simulink model "Test3"  (R2017b)
settings: Solver=ode23tb  StartTime=0.0  StopTime=6  MaxStep=1e-4  RelTol=1e-3
libraries: powerlib x4
settings Model: Creator=80573  LastModifiedBy=80573

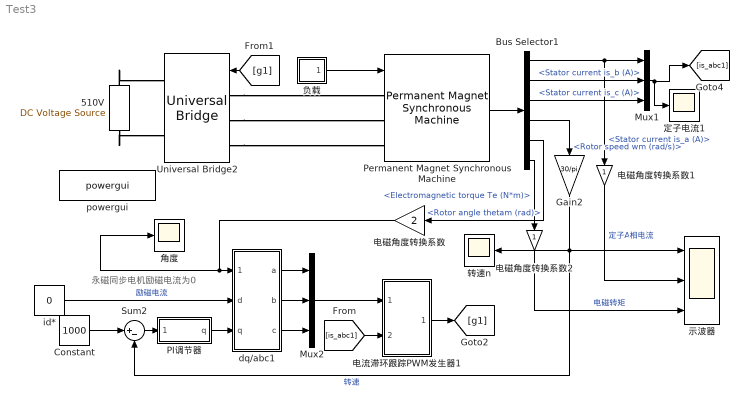
== system Test3 ==
  note: 永磁同步电机励磁电流为0
  510V : powerlib/Electrical Sources/DC Voltage Source  Amplitude=800  Measurements=None
  Bus Selector1 : BusSelector  OutputSignals=Stator current is_a (A),Stator current is_b (A),Stator current is_c (A),Rotor speed wm (rad/s),Rotor angle thetam (rad),Electromagnetic torque Te (N*m)
  Constant : Constant  Value=1000
  Gain2 : Gain  Gain=30/pi
  Mux1 : Mux  Inputs=3
  Mux2 : Mux  Inputs=3
  PI调节器 : Subsystem
  Permanent Magnet Synchronous Machine : powerlib/Machines/Permanent Magnet Synchronous Machine  NbPhases=3  FluxDistribution=Sinusoidal  RotorType=Salient-pole  MechanicalLoad=Torque Tm  PresetModel=No  ShowDetailedParameters=on  MeasurementBus=off  Resistance=0.00275  Inductance=8.5e-3  dqInductances=[0.000085 0.000085]  La=0.02682  MachineConstant=Flux linkage established by magnets (V.s)  Flux=1  VoltageCst=362.7599  TorqueCst=3  Flat=120  Mechanical=[1 0.008 2 0]  PolePairs=2  InitialConditions=[0,0, 0,0]  InitialConditions5ph=[0 0 0 0 0 0]  TsPowergui=0  TsBlock=-1  RefAngle=Aligned with phase A axis (original Park)
      settings: SourceProductName=Simscape Power Systems
  Sum2 : Sum  Inputs=|+-
  Universal Bridge2 : powerlib/Power Electronics/Universal Bridge  Arms=3  SnubberResistance=1e5  SnubberCapacitance=inf  Device=IGBT / Diodes  Ron=1e-3  Lon=0  ForwardVoltages="[  0  0  ]"  ForwardVoltage=0  GTOparameters=[ 10e-6 , 20e-6 ]  IGBTparameters=[ 1e-6 , 2e-6 ]  Measurements=None  Measurements_2=None  converterType=Rectifier
  dq/abc1 : Subsystem
  id* : Constant  Value=0
  powergui : powerlib/powergui  SimulationMode=Discrete  SampleTime=0.00001  frequency=50  Iterations=50  frequencyindice=0  Pbase=100e6  ErrMax=1e-4  UnitsV=kV  UnitsW=MW  buscounter=0  FunctionMessages=off  echomessages=off  EnableUseOfTLC=off  CurrentSourceSwitches=off  DisableSnubberDevices=off  DisableRonSwitches=off  DisableVfSwitches=off  DisplayEquations=off  SolverType=Tustin/Backward Euler (TBE)  Interpol=off  ExternalGateDelay=off  methode=off  Ts=100  x0status=zero  SPID=on  SwTol=0  HookPort=off  RestoreLinks=warning  ResistiveCurrentMeasurement=off  Frange=[0:2:500]  Ylog=off  Xlog=on  ShowGrid=off  save=off  variable=ZData  structure=0  ZoomFFT=on  StartTime=0.0  cycles=1  DisplayStyle=1  fundamental=60  FreqAxis=off  MaxFrequency=1000  frequencyindicesteady=1  RmsSteady=1  display=off
  定子电流1 : Scope
  电流滞环跟踪PWM发生器1 : Subsystem
  电磁角度转换系数 : Gain  Gain=2
  电磁角度转换系数1 : Gain
  电磁角度转换系数2 : Gain
  示波器 : Scope  NumInputPorts=3
  角度 : Scope
  负载 : Subsystem
  转速n : Scope
  wires:
  Bus Selector1/3 -> Mux1/3  "<Stator current is_c (A)>"
  Mux1/1 -> [is_abc1], 定子电流1/1
  Bus Selector1/5 -> 电磁角度转换系数/1  "<Rotor angle thetam (rad)>"
  dq/abc1/3(c) -> Mux2/3
  [is_abc1] -> 电流滞环跟踪PWM发生器1/2(Iabc)
  电流滞环跟踪PWM发生器1/1(pulse) -> [g1]
  PI调节器/1(q) -> dq/abc1/3(q)
  Gain2/1 -> 示波器/1, Sum2/2, 转速n/1  "转速"
  [g1] -> Universal Bridge2/1
  Bus Selector1/6 -> 电磁角度转换系数2/1  "<Electromagnetic torque Te (N*m)>"
  dq/abc1/2(b) -> Mux2/2
  电磁角度转换系数2/1 -> 示波器/3  "电磁转矩"
  电磁角度转换系数1/1 -> 示波器/2  "定子A相电流"
  Mux2/1 -> 电流滞环跟踪PWM发生器1/1(Iabc*)
  Bus Selector1/1 -> Mux1/1, 电磁角度转换系数1/1  "<Stator current is_a (A)>"
  Permanent Magnet Synchronous Machine/1 -> Bus Selector1/1
  id*/1 -> dq/abc1/2(d)  "励磁电流"
  电磁角度转换系数/1 -> 角度/1, dq/abc1/1(theta)
  Bus Selector1/4 -> Gain2/1  "<Rotor speed wm (rad/s)>"
  Sum2/1 -> PI调节器/1("  ")
  负载/1(TL) -> Permanent Magnet Synchronous Machine/1
  Constant/1 -> Sum2/1
  dq/abc1/1(a) -> Mux2/1
  Bus Selector1/2 -> Mux1/2  "<Stator current is_b (A)>"
  connections:
  510V/RConn1 -- Universal Bridge2/RConn1
  Universal Bridge2/LConn1 -- Permanent Magnet Synchronous Machine/LConn1
  Universal Bridge2/LConn3 -- Permanent Magnet Synchronous Machine/LConn3
  510V/LConn1 -- Universal Bridge2/RConn2
  Universal Bridge2/LConn2 -- Permanent Magnet Synchronous Machine/LConn2

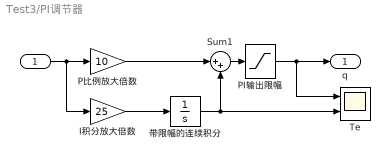
== system Test3/PI调节器 ==
  "  " : Inport
  I积分放大倍数 : Gain  Gain=25
  PI输出限幅 : Saturate  UpperLimit=500  LowerLimit=-500
  P比例放大倍数 : Gain  Gain=10
  Sum1 : Sum  Inputs=|++
  Te : Scope  NumInputPorts=2
  带限幅的连续积分 : Integrator  LimitOutput=on  UpperSaturationLimit=510  LowerSaturationLimit=-510
  q : Outport
  wires:
  Sum1/1 -> PI输出限幅/1
  PI输出限幅/1 -> q/1, Te/1
  P比例放大倍数/1 -> Sum1/1
  I积分放大倍数/1 -> 带限幅的连续积分/1
  带限幅的连续积分/1 -> Te/2, Sum1/2
  "  "/1 -> I积分放大倍数/1, P比例放大倍数/1

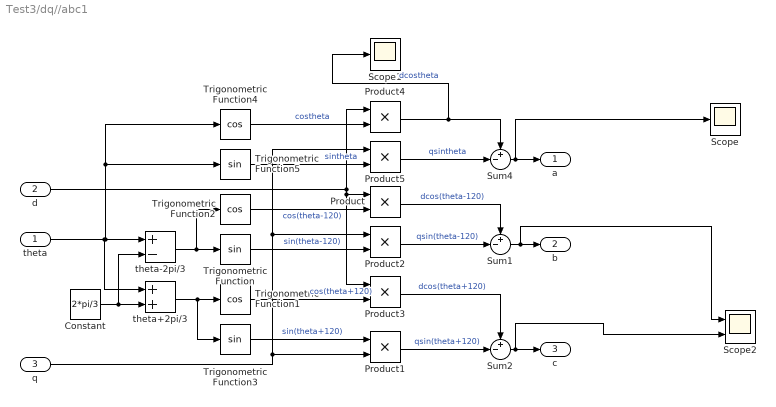
== system Test3/dq//abc1 ==
  theta : Inport
  d : Inport  Port=2
  q : Inport  Port=3
  Constant : Constant  Value=2*pi/3
  Product{,1..5} (6 alike) : Product
  Scope : Scope
  Scope1 : Scope
  Scope2 : Scope  NumInputPorts=2
  Sum1 : Sum  Inputs=+-|
  Sum2 : Sum  Inputs=+-|
  Sum4 : Sum  Inputs=+-|
  Trigonometric Function : Trigonometry
  Trigonometric Function1 : Trigonometry  Operator=cos
  Trigonometric Function2 : Trigonometry  Operator=cos
  Trigonometric Function3 : Trigonometry
  Trigonometric Function4 : Trigonometry  Operator=cos
  Trigonometric Function5 : Trigonometry
  theta+2pi/3 : Sum
  theta-2pi/3 : Sum  Inputs=+-
  a : Outport
  b : Outport  Port=2
  c : Outport  Port=3
  wires:
  Trigonometric Function5/1 -> Product5/2  "sintheta"
  Product/1 -> Sum1/1  "dcos(theta-120)"
  Trigonometric Function1/1 -> Product3/2  "cos(theta+120)"
  Product3/1 -> Sum2/1  "dcos(theta+120)"
  d/1 -> Product/1, Product3/1, Product4/1
  Constant/1 -> theta+2pi/3/2, theta-2pi/3/2
  theta/1 -> Trigonometric Function4/1, Trigonometric Function5/1, theta-2pi/3/1, theta+2pi/3/1
  theta+2pi/3/1 -> Trigonometric Function3/1, Trigonometric Function1/1
  q/1 -> Product5/1, Product2/1, Product1/2
  Trigonometric Function/1 -> Product2/2  "sin(theta-120)"
  Product4/1 -> Scope1/1, Sum4/1  "dcostheta"
  Product5/1 -> Sum4/2  "qsintheta"
  theta-2pi/3/1 -> Trigonometric Function2/1, Trigonometric Function/1
  Product1/1 -> Sum2/2  "qsin(theta+120)"
  Trigonometric Function2/1 -> Product/2  "cos(theta-120)"
  Sum4/1 -> Scope/1, a/1
  Sum1/1 -> Scope2/1, b/1
  Trigonometric Function4/1 -> Product4/2  "costheta"
  Trigonometric Function3/1 -> Product1/1  "sin(theta+120)"
  Product2/1 -> Sum1/2  "qsin(theta-120)"
  Sum2/1 -> Scope2/2, c/1

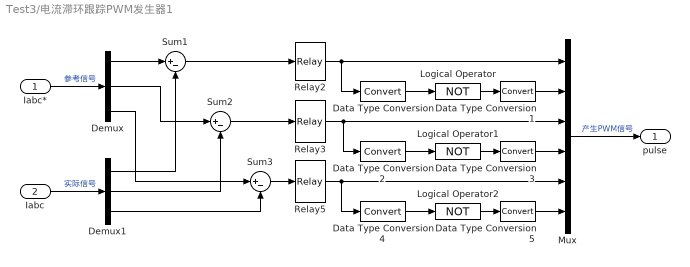
== system Test3/电流滞环跟踪PWM发生器1 ==
  Iabc* : Inport
  Iabc : Inport  Port=2
  Data Type Conversion{,1..5} (6 alike) : DataTypeConversion
  Demux : Demux  Outputs=3
  Demux1 : Demux  Outputs=3
  Logical Operator : Logic  Operator=NOT  Inputs=1  AllPortsSameDT=off
  Logical Operator1 : Logic  Operator=NOT  Inputs=1  AllPortsSameDT=off
  Logical Operator2 : Logic  Operator=NOT  Inputs=1  AllPortsSameDT=off
  Mux : Mux  Inputs=6
  Relay2 : Relay  OnSwitchValue=0.1  OffSwitchValue=-0.1  ZeroCross=off
  Relay3 : Relay  OnSwitchValue=0.1  OffSwitchValue=-0.1  ZeroCross=off
  Relay5 : Relay  OnSwitchValue=0.1  OffSwitchValue=-0.1  ZeroCross=off
  Sum1 : Sum  Inputs=|+-
  Sum2 : Sum  Inputs=|+-
  Sum3 : Sum  Inputs=|+-
  pulse : Outport
  wires:
  Relay2/1 -> Data Type Conversion/1, Mux/1
  Data Type Conversion/1 -> Logical Operator/1
  Logical Operator/1 -> Data Type Conversion1/1
  Data Type Conversion1/1 -> Mux/2
  Mux/1 -> pulse/1  "产生PWM信号"
  Sum1/1 -> Relay2/1
  Demux/1 -> Sum1/1
  Demux1/3 -> Sum3/2
  Iabc/1 -> Demux1/1  "实际信号"
  Iabc*/1 -> Demux/1  "参考信号"
  Sum2/1 -> Relay3/1
  Logical Operator1/1 -> Data Type Conversion3/1
  Data Type Conversion3/1 -> Mux/4
  Data Type Conversion2/1 -> Logical Operator1/1
  Relay3/1 -> Data Type Conversion2/1, Mux/3
  Logical Operator2/1 -> Data Type Conversion5/1
  Data Type Conversion5/1 -> Mux/6
  Data Type Conversion4/1 -> Logical Operator2/1
  Relay5/1 -> Data Type Conversion4/1, Mux/5
  Sum3/1 -> Relay5/1
  Demux/2 -> Sum2/1
  Demux1/1 -> Sum1/2
  Demux1/2 -> Sum2/2
  Demux/3 -> Sum3/1

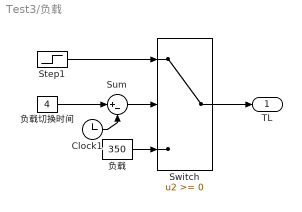
== system Test3/负载 ==
  Clock1 : Clock
  Step1 : Step  Time=2  Before=200  After=500  SampleTime=0
  Sum : Sum  Inputs=|+-
  Switch : Switch
  负载 : Constant  Value=350
  负载切换时间 : Constant  Value=4
  TL : Outport
  wires:
  Clock1/1 -> Sum/2
  Switch/1 -> TL/1
  Sum/1 -> Switch/2
  负载/1 -> Switch/3
  负载切换时间/1 -> Sum/1
  Step1/1 -> Switch/1
